simulink model "sensor_test_bench"  (R2022a)
settings: Solver=VariableStepAuto  StartTime=0.0  StopTime=1  RelTol=1e-3
InitFcn:
  | ELEN90064_Project_Parameters
values from neighbouring files (symbols this model uses):
  absolute_encoder_counts_per_revolution = 4096    [ELEN90064_Project_Parameters.m]
  gyro_sigma_drift = deg2rad(5)    [ELEN90064_Project_Parameters.m]
  potentiometer_linearity_percent = 20    [ELEN90064_Project_Parameters.m]
  tachometer_counts_per_revolution = 2048    [ELEN90064_Project_Parameters.m]
  tachometer_output_frequency = 50    [ELEN90064_Project_Parameters.m]
  theta_l_init = deg2rad(0)    [ELEN90064_Project_Parameters.m]
  theta_m_init = deg2rad(0)    [ELEN90064_Project_Parameters.m]
  thetadot_m_init = deg2rad(0)    [ELEN90064_Project_Parameters.m]
  vision_fps = 50    [ELEN90064_Project_Parameters.m]
libraries: simulink x1
settings Model: Creator=pbeuchat  LastModifiedBy=yang
settings SolverCC: AlgebraicLoopSolver=TrustRegion
settings DebuggingCC: UnconnectedInputMsg=warning  UnconnectedOutputMsg=warning  UnconnectedLineMsg=warning  SFMachineParentedDataDiag=warning
settings RTWCC: DLArmComputeVersion=19.05

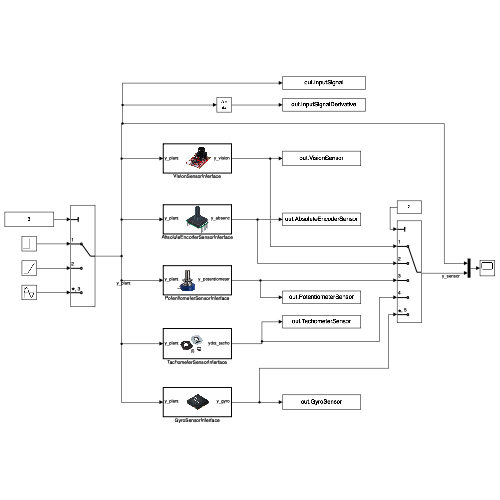
[thumbnail: Simulink's stored preview of the top-level diagram]
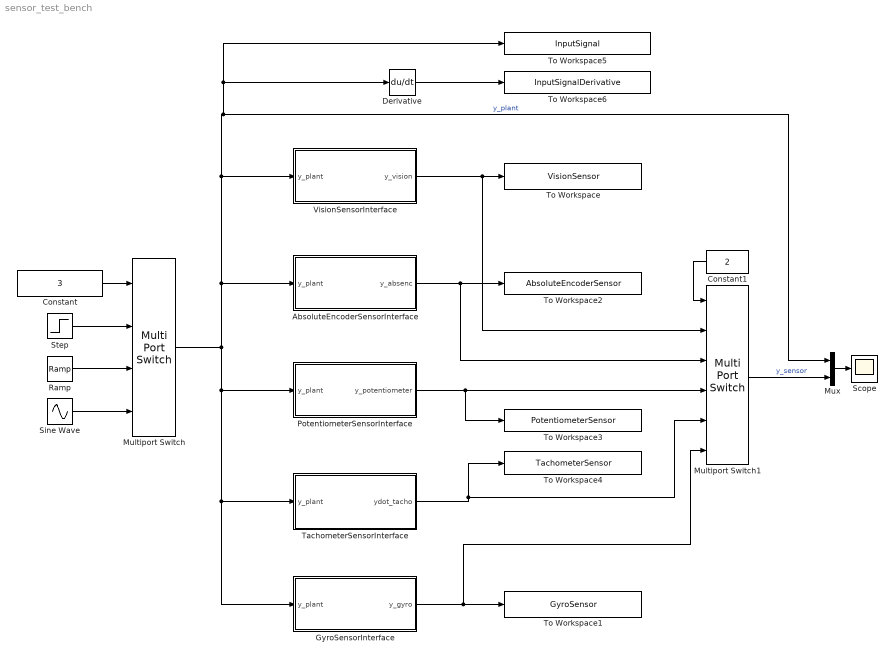
== system sensor_test_bench ==
  AbsoluteEncoderSensorInterface : Subsystem  TreatAsAtomicUnit=on
      mask Display: image('$imagefile'); % Use "Edit Image" on toolstrip to change.
  Constant : Constant  Value=3
  Constant1 : Constant  Value=2
  Derivative : Derivative
  GyroSensorInterface : Subsystem  TreatAsAtomicUnit=on
      mask Display: image('$imagefile'); % Use "Edit Image" on toolstrip to change.
  Multiport Switch : MultiPortSwitch  SaturateOnIntegerOverflow=off  InputSameDT=off
  Multiport Switch1 : MultiPortSwitch  Inputs=5  SaturateOnIntegerOverflow=off  InputSameDT=off
  Mux : Mux  Inputs=2
  PotentiometerSensorInterface : Subsystem  TreatAsAtomicUnit=on
      mask Display: image('$imagefile'); % Use "Edit Image" on toolstrip to change.
  Ramp : simulink/Sources/Ramp  slope=deg2rad(90)  start=0.1  InitialOutput=theta_l_init
  Scope : Scope
  Sine Wave : Sin  Amplitude=deg2rad(90)  Frequency=4*pi  SampleTime=0
  Step : Step  Time=0.1  Before=theta_l_init  After=deg2rad(90)  SampleTime=0
  TachometerSensorInterface : Subsystem  TreatAsAtomicUnit=on
      mask Display: image('$imagefile'); % Use "Edit Image" on toolstrip to change.
  To Workspace : ToWorkspace  VariableName=VisionSensor  SaveFormat=Timeseries  SampleTime=1/1000
  To Workspace1 : ToWorkspace  VariableName=GyroSensor  SaveFormat=Timeseries  SampleTime=1/1000
  To Workspace2 : ToWorkspace  VariableName=AbsoluteEncoderSensor  SaveFormat=Timeseries  SampleTime=1/1000
  To Workspace3 : ToWorkspace  VariableName=PotentiometerSensor  SaveFormat=Timeseries  SampleTime=1/1000
  To Workspace4 : ToWorkspace  VariableName=TachometerSensor  SaveFormat=Timeseries  SampleTime=1/1000
  To Workspace5 : ToWorkspace  VariableName=InputSignal  SaveFormat=Timeseries  SampleTime=1/1000
  To Workspace6 : ToWorkspace  VariableName=InputSignalDerivative  SaveFormat=Timeseries  SampleTime=1/1000
  VisionSensorInterface : Subsystem  TreatAsAtomicUnit=on
      mask Display: image('$imagefile'); % Use "Edit Image" on toolstrip to change.
  wires:
  Ramp/1 -> Multiport Switch/3
  Step/1 -> Multiport Switch/2
  Sine Wave/1 -> Multiport Switch/4
  Constant/1 -> Multiport Switch/1
  Multiport Switch/1 -> AbsoluteEncoderSensorInterface/1(y_plant), VisionSensorInterface/1(y_plant), Derivative/1, To Workspace5/1, Mux/1, GyroSensorInterface/1(y_plant), TachometerSensorInterface/1(y_plant), PotentiometerSensorInterface/1(y_plant)  "y_plant"
  VisionSensorInterface/1(y_vision) -> Multiport Switch1/2, To Workspace/1
  Multiport Switch1/1 -> Mux/2  "y_sensor"
  Mux/1 -> Scope/1
  Constant1/1 -> Multiport Switch1/1
  GyroSensorInterface/1(y_gyro) -> Multiport Switch1/6, To Workspace1/1
  AbsoluteEncoderSensorInterface/1(y_absenc) -> Multiport Switch1/3, To Workspace2/1
  PotentiometerSensorInterface/1(y_potentiometer) -> To Workspace3/1, Multiport Switch1/4
  TachometerSensorInterface/1(ydot_tacho) -> To Workspace4/1, Multiport Switch1/5
  Derivative/1 -> To Workspace6/1

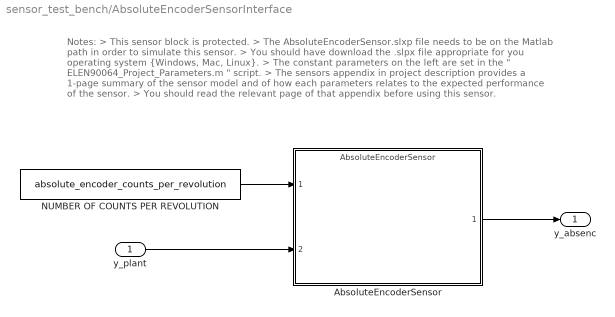
== system sensor_test_bench/AbsoluteEncoderSensorInterface ==
  note: Notes:
      | > This sensor block is protected.
      | > The AbsoluteEncoderSensor.slxp file needs to be on the Matlab path in order to simulate this sensor.
      | > You should have download the .slpx file appropriate for you operating system {Windows, Mac, Linux}.
      | > The constant parameters on the left are set in the " ELEN90064_Project_Parameters.m " script.
      | > The sensors appendix in project description provides a 1-page summary of the sensor model and of how each parameters relates to the expected performance of the sensor.
      | > You should read the relevant page of that appendix before using this sensor.
  y_plant : Inport
  AbsoluteEncoderSensor : ModelReference  ModelNameDialog=AbsoluteEncoderSensor.slxp  ModelReferenceVersion=1.16  CopyOfModelProtected=on
  NUMBER OF COUNTS PER REVOLUTION : Constant  Value=absolute_encoder_counts_per_revolution
  y_absenc : Outport
  wires:
  NUMBER OF COUNTS PER REVOLUTION/1 -> AbsoluteEncoderSensor/1
  y_plant/1 -> AbsoluteEncoderSensor/2
  AbsoluteEncoderSensor/1 -> y_absenc/1

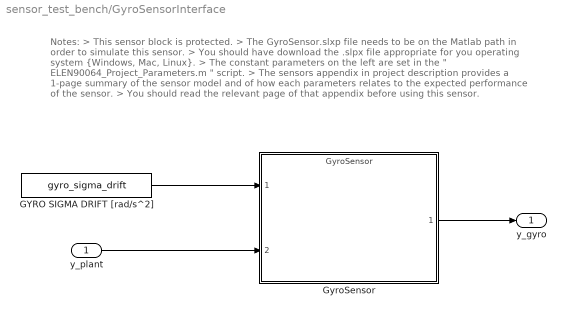
== system sensor_test_bench/GyroSensorInterface ==
  note: Notes:
      | > This sensor block is protected.
      | > The GyroSensor.slxp file needs to be on the Matlab path in order to simulate this sensor.
      | > You should have download the .slpx file appropriate for you operating system {Windows, Mac, Linux}.
      | > The constant parameters on the left are set in the " ELEN90064_Project_Parameters.m " script.
      | > The sensors appendix in project description provides a 1-page summary of the sensor model and of how each parameters relates to the expected performance of the sensor.
      | > You should read the relevant page of that appendix before using this sensor.
  y_plant : Inport
  GYRO SIGMA DRIFT [rad/s^2] : Constant  Value=gyro_sigma_drift
  GyroSensor : ModelReference  ModelNameDialog=GyroSensor.slxp  ModelReferenceVersion=1.18  CopyOfModelProtected=on
  y_gyro : Outport
  wires:
  GYRO SIGMA DRIFT [rad/s^2]/1 -> GyroSensor/1
  y_plant/1 -> GyroSensor/2
  GyroSensor/1 -> y_gyro/1

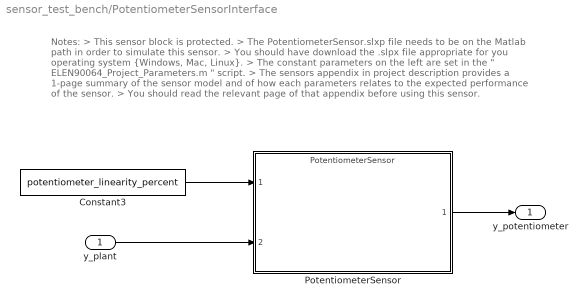
== system sensor_test_bench/PotentiometerSensorInterface ==
  note: Notes:
      | > This sensor block is protected.
      | > The PotentiometerSensor.slxp file needs to be on the Matlab path in order to simulate this sensor.
      | > You should have download the .slpx file appropriate for you operating system {Windows, Mac, Linux}.
      | > The constant parameters on the left are set in the " ELEN90064_Project_Parameters.m " script.
      | > The sensors appendix in project description provides a 1-page summary of the sensor model and of how each parameters relates to the expected performance of the sensor.
      | > You should read the relevant page of that appendix before using this sensor.
  y_plant : Inport
  Constant3 : Constant  Value=potentiometer_linearity_percent
  PotentiometerSensor : ModelReference  ModelNameDialog=PotentiometerSensor.slxp  ModelReferenceVersion=1.21  CopyOfModelProtected=on
  y_potentiometer : Outport
  wires:
  y_plant/1 -> PotentiometerSensor/2
  Constant3/1 -> PotentiometerSensor/1
  PotentiometerSensor/1 -> y_potentiometer/1

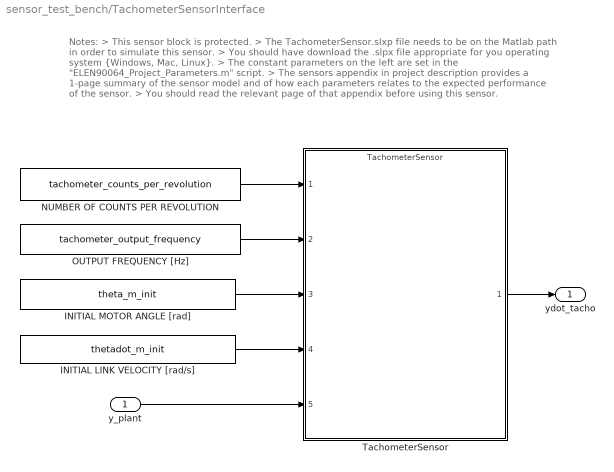
== system sensor_test_bench/TachometerSensorInterface ==
  note: Notes:
      | > This sensor block is protected.
      | > The TachometerSensor.slxp file needs to be on the Matlab path in order to simulate this sensor.
      | > You should have download the .slpx file appropriate for you operating system {Windows, Mac, Linux}.
      | > The constant parameters on the left are set in the "ELEN90064_Project_Parameters.m" script.
      | > The sensors appendix in project description provides a 1-page summary of the sensor model and of how each parameters relates to the expected performance of the sensor.
      | > You should read the relevant page of that appendix before using this sensor.
  y_plant : Inport
  INITIAL LINK VELOCITY [rad/s] : Constant  Value=thetadot_m_init
  INITIAL MOTOR ANGLE [rad] : Constant  Value=theta_m_init
  NUMBER OF COUNTS PER REVOLUTION : Constant  Value=tachometer_counts_per_revolution
  OUTPUT FREQUENCY [Hz] : Constant  Value=tachometer_output_frequency
  TachometerSensor : ModelReference  ModelNameDialog=TachometerSensor.slxp  ModelReferenceVersion=1.31  CopyOfModelProtected=on
  ydot_tacho : Outport
  wires:
  INITIAL MOTOR ANGLE [rad]/1 -> TachometerSensor/3
  INITIAL LINK VELOCITY [rad/s]/1 -> TachometerSensor/4
  y_plant/1 -> TachometerSensor/5
  NUMBER OF COUNTS PER REVOLUTION/1 -> TachometerSensor/1
  OUTPUT FREQUENCY [Hz]/1 -> TachometerSensor/2
  TachometerSensor/1 -> ydot_tacho/1

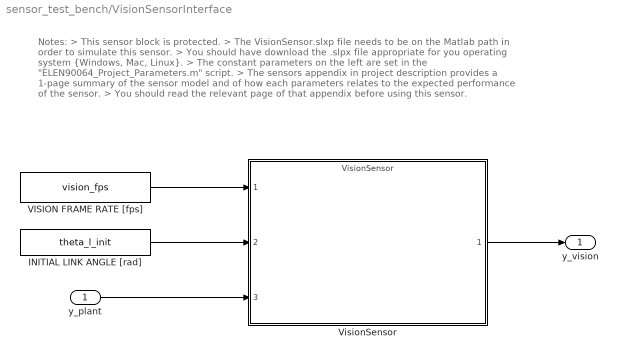
== system sensor_test_bench/VisionSensorInterface ==
  note: Notes:
      | > This sensor block is protected.
      | > The VisionSensor.slxp file needs to be on the Matlab path in order to simulate this sensor.
      | > You should have download the .slpx file appropriate for you operating system {Windows, Mac, Linux}.
      | > The constant parameters on the left are set in the "ELEN90064_Project_Parameters.m" script.
      | > The sensors appendix in project description provides a 1-page summary of the sensor model and of how each parameters relates to the expected performance of the sensor.
      | > You should read the relevant page of that appendix before using this sensor.
  y_plant : Inport
  INITIAL LINK ANGLE [rad] : Constant  Value=theta_l_init
  VISION FRAME RATE [fps] : Constant  Value=vision_fps
  VisionSensor : ModelReference  ModelNameDialog=VisionSensor.slxp  ModelReferenceVersion=1.19  CopyOfModelProtected=on
  y_vision : Outport
  wires:
  VISION FRAME RATE [fps]/1 -> VisionSensor/1
  INITIAL LINK ANGLE [rad]/1 -> VisionSensor/2
  y_plant/1 -> VisionSensor/3
  VisionSensor/1 -> y_vision/1
